simulink model "model"  (R2019b)
settings: Solver=ode3  StartTime=0.0  StopTime=12  FixedStep=0.01  RelTol=1e-3
values from neighbouring files (symbols this model uses):
  A = [0 1;0 0]    [init.m]
  B = [0;1/J]    [init.m]
  C = [1 0;0 1]    [init.m]
  csys = c2d(sys, 0.01)    [init.m]
  D = [0;0]    [init.m]
  K = acker(A,B,[p1, p2])    [init.m]
  K_ = acker(A_,B_,[p1, p2, -7.8])    [init.m]
settings Model: Creator=Daniel  LastModifiedBy=Daniel

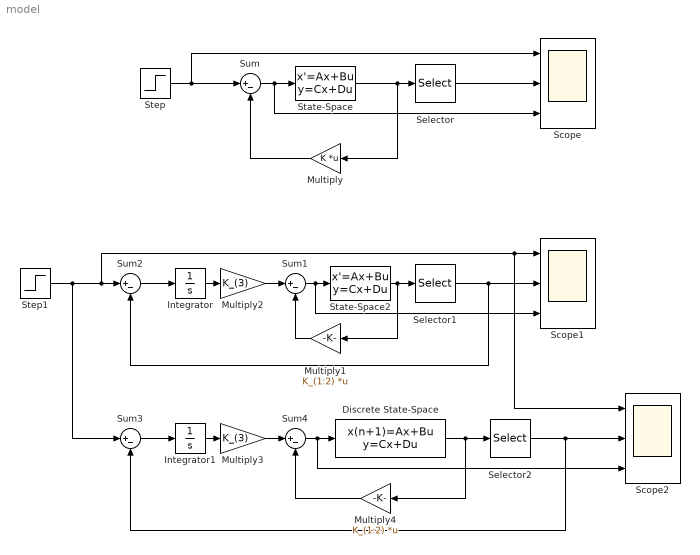
== system model ==
  Discrete State-Space : DiscreteStateSpace  A=csys.A  B=csys.B  C=csys.C  D=csys.D  SampleTime=-1
  Integrator : Integrator
  Integrator1 : Integrator
  Multiply : Gain  Gain=K  Multiplication=Matrix(K*u)
  Multiply1 : Gain  Gain=K_(1:2)  Multiplication=Matrix(K*u)
  Multiply2 : Gain  Gain=K_(3)
  Multiply3 : Gain  Gain=K_(3)
  Multiply4 : Gain  Gain=K_(1:2)  Multiplication=Matrix(K*u)
  Scope : Scope  NumInputPorts=3
  Scope1 : Scope  NumInputPorts=3
  Scope2 : Scope  NumInputPorts=3
  Selector : Selector  InputPortWidth=2  IndexOptions=Index vector (dialog)  Indices=1  OutputSizes=1
  Selector1 : Selector  InputPortWidth=2  IndexOptions=Index vector (dialog)  Indices=1  OutputSizes=1
  Selector2 : Selector  InputPortWidth=2  IndexOptions=Index vector (dialog)  Indices=1  OutputSizes=1
  State-Space : StateSpace  A=A  B=B  C=C  D=D  InitialCondition=0
  State-Space2 : StateSpace  A=A  B=B  C=C  D=D  InitialCondition=0
  Step : Step  SampleTime=0
  Step1 : Step  SampleTime=0
  Sum{,1..4} (5 alike) : Sum  Inputs=|+-
  wires:
  State-Space/1 -> Selector/1, Multiply/1
  Step/1 -> Scope/1, Sum/1
  Sum/1 -> Scope/3, State-Space/1
  Multiply/1 -> Sum/2
  Selector/1 -> Scope/2
  Selector1/1 -> Sum2/2, Scope1/2
  Step1/1 -> Sum3/1, Sum2/1, Scope2/1, Scope1/1
  State-Space2/1 -> Selector1/1, Multiply1/1
  Sum2/1 -> Integrator/1
  Integrator/1 -> Multiply2/1
  Multiply2/1 -> Sum1/1
  Sum1/1 -> Scope1/3, State-Space2/1
  Multiply1/1 -> Sum1/2
  Discrete State-Space/1 -> Multiply4/1, Selector2/1
  Selector2/1 -> Sum3/2, Scope2/2
  Integrator1/1 -> Multiply3/1
  Sum3/1 -> Integrator1/1
  Multiply3/1 -> Sum4/1
  Sum4/1 -> Scope2/3, Discrete State-Space/1
  Multiply4/1 -> Sum4/2
